simulink model "PiFace_Ctrl_Modbus_exec"  (Simulink 3.00)
libraries: execlib x6

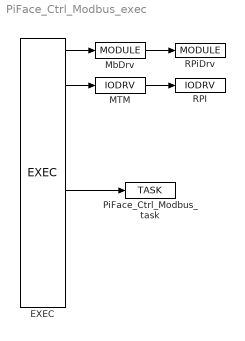
== system PiFace_Ctrl_Modbus_exec ==
  EXEC : execlib/EXEC  target=PC - Linux  tick=0.05  ntick0=2  ntick1=50  ntick2=100  ntick3=1200  pri0=5  pri1=9  pri2=13  pri3=18
  MTM : execlib/IODRV  module=MbDrv  classname=MtmDrv  cfgname=PiFace_Ctrl_Modbus_cfg.rio  factor=10  stack=10240  pri=3  timer=off
  MbDrv : execlib/MODULE
  PiFace_Ctrl_Modbus_task : execlib/TASK  factor=1  start=1  stop=2  stack=10240  MDLOPEN=on
  RPI : execlib/IODRV  module=RPiDrv  classname=RPiDrv  factor=1  stack=10240  pri=3  timer=off
  RPiDrv : execlib/MODULE
  wires:
  EXEC/1 -> MbDrv/1
  EXEC/2 -> MTM/1
  EXEC/5 -> PiFace_Ctrl_Modbus_task/1
  MTM/1 -> RPI/1
  MbDrv/1 -> RPiDrv/1
